simulink model "pedal_req_02"  (R2018b)
settings: Solver=FixedStepDiscrete  StartTime=0.0  StopTime=10.0  RelTol=1e-3
libraries: simulink x1
settings Model: Creator=yangbo  LastModifiedBy=yangbo_91
settings OptimizationCC: DefaultParameterBehavior=Inlined  EnhancedBackFolding=on  PassReuseOutputArgsAs=Individual arguments  OptimizeBlockOrder=speed  DifferentSizesBufferReuse=on  OptimizationCustomize=off
settings DebuggingCC: ParameterTunabilityLossMsg=error
settings SFSimCC: MATLABDynamicMemAlloc=off
settings RTWCC: SystemTargetFile=ert.tlc  TemplateMakefile=ert_default_tmf  GenerateReport=on  IncludeHyperlinkInReport=on  LaunchReport=on  GenerateTraceInfo=on  GenerateTraceReport=on  GenerateTraceReportSl=on  GenerateTraceReportSf=on  GenerateTraceReportEml=on
settings CodeAppCC: ForceParamTrailComments=on  IgnoreCustomStorageClasses=off  OperatorAnnotations=on  SimulinkDataObjDesc=on  SFDataObjDesc=on  InsertBlockDesc=on
settings ERTTargetCC: TargetLangStandard=C99 (ISO)  GenerateSampleERTMain=on  InlinedParameterPlacement=NonHierarchical  ERTCustomFileTemplate=example_file_process.tlc

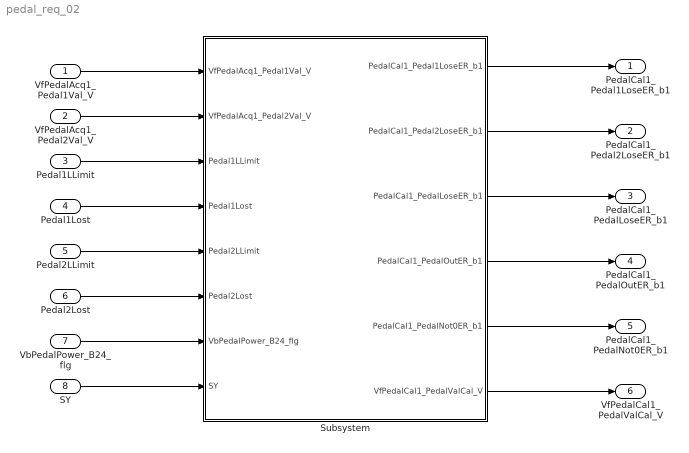
== system pedal_req_02 ==
  VfPedalAcq1_Pedal1Val_V : Inport
  VfPedalAcq1_Pedal2Val_V : Inport  Port=2
  Pedal1LLimit : Inport  Port=3
  Pedal1Lost : Inport  Port=4
  Pedal2LLimit : Inport  Port=5
  Pedal2Lost : Inport  Port=6
  VbPedalPower_B24_flg : Inport  Port=7
  SY : Inport  Port=8
  Subsystem : Subsystem  TreatAsAtomicUnit=on
  PedalCal1_Pedal1LoseER_b1 : Outport
  PedalCal1_Pedal2LoseER_b1 : Outport  Port=2
  PedalCal1_PedalLoseER_b1 : Outport  Port=3
  PedalCal1_PedalOutER_b1 : Outport  Port=4
  PedalCal1_PedalNot0ER_b1 : Outport  Port=5
  VfPedalCal1_PedalValCal_V : Outport  Port=6
  wires:
  VfPedalAcq1_Pedal1Val_V/1 -> Subsystem/1(VfPedalAcq1_Pedal1Val_V)
  VfPedalAcq1_Pedal2Val_V/1 -> Subsystem/2(VfPedalAcq1_Pedal2Val_V)
  Pedal1LLimit/1 -> Subsystem/3(Pedal1LLimit)
  Pedal1Lost/1 -> Subsystem/4(Pedal1Lost)
  Pedal2LLimit/1 -> Subsystem/5(Pedal2LLimit)
  Pedal2Lost/1 -> Subsystem/6(Pedal2Lost)
  VbPedalPower_B24_flg/1 -> Subsystem/7(VbPedalPower_B24_flg)
  SY/1 -> Subsystem/8(SY)
  Subsystem/1(PedalCal1_Pedal1LoseER_b1) -> PedalCal1_Pedal1LoseER_b1/1
  Subsystem/2(PedalCal1_Pedal2LoseER_b1) -> PedalCal1_Pedal2LoseER_b1/1
  Subsystem/3(PedalCal1_PedalLoseER_b1) -> PedalCal1_PedalLoseER_b1/1
  Subsystem/4(PedalCal1_PedalOutER_b1) -> PedalCal1_PedalOutER_b1/1
  Subsystem/5(PedalCal1_PedalNot0ER_b1) -> PedalCal1_PedalNot0ER_b1/1
  Subsystem/6(VfPedalCal1_PedalValCal_V) -> VfPedalCal1_PedalValCal_V/1

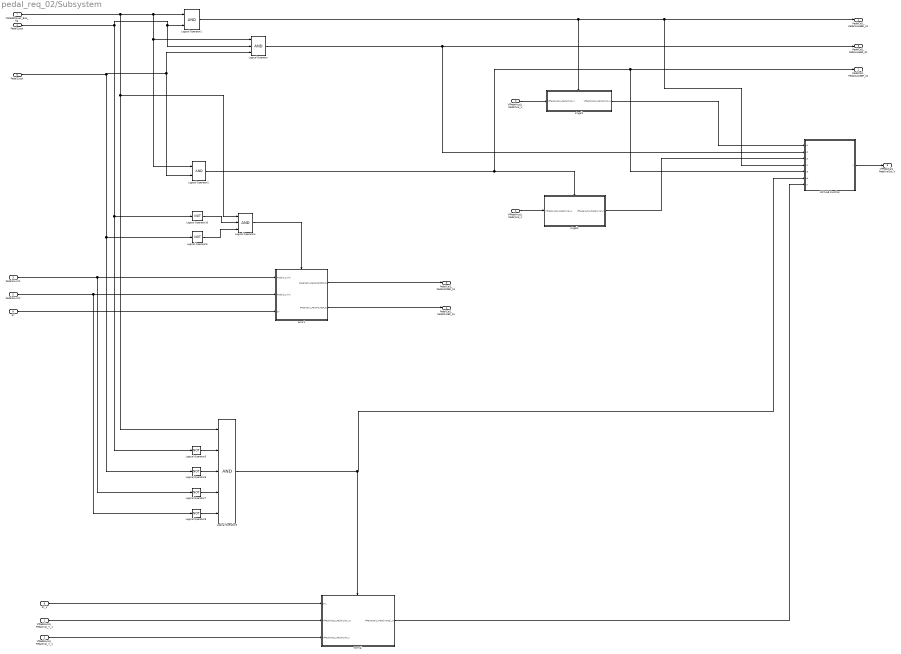
== system pedal_req_02/Subsystem ==
  VfPedalAcq1_Pedal1Val_V : Inport
  VfPedalAcq1_Pedal2Val_V : Inport  Port=2
  Pedal1LLimit : Inport  Port=3
  Pedal1Lost : Inport  Port=4
  Pedal2LLimit : Inport  Port=5
  Pedal2Lost : Inport  Port=6
  VbPedalPower_B24_flg : Inport  Port=7
  SY : Inport  Port=8
  Logical Operator : Logic  Inputs=3  AllPortsSameDT=off  OutDataTypeStr=boolean
  Logical Operator1 : Logic  AllPortsSameDT=off  OutDataTypeStr=boolean
  Logical Operator10 : Logic  Operator=NOT  Inputs=3  AllPortsSameDT=off  OutDataTypeStr=boolean
  Logical Operator2 : Logic  AllPortsSameDT=off  OutDataTypeStr=boolean
  Logical Operator3 : Logic  Inputs=5  AllPortsSameDT=off  OutDataTypeStr=boolean
  Logical Operator4 : Logic  Inputs=3  AllPortsSameDT=off  OutDataTypeStr=boolean
  Logical Operator{5..8} (4 alike) : Logic  Operator=NOT  AllPortsSameDT=off  OutDataTypeStr=boolean
  Logical Operator9 : Logic  Operator=NOT  Inputs=3  AllPortsSameDT=off  OutDataTypeStr=boolean
  MATLAB Function : MATLAB Function  TreatAsAtomicUnit=on
  SY_1 : InportShadow  Port=8
  VfPedalAcq1_Pedal1Val_V_1 : InportShadow
  VfPedalAcq1_Pedal2Val_V_1 : InportShadow  Port=2
  error1 : Subsystem  TreatAsAtomicUnit=on
  normal : Subsystem  TreatAsAtomicUnit=on
  singal1 : Subsystem  TreatAsAtomicUnit=on
  singal2 : Subsystem  TreatAsAtomicUnit=on
  PedalCal1_Pedal1LoseER_b1 : Outport
  PedalCal1_Pedal2LoseER_b1 : Outport  Port=2
  PedalCal1_PedalLoseER_b1 : Outport  Port=3
  PedalCal1_PedalOutER_b1 : Outport  Port=4
  PedalCal1_PedalNot0ER_b1 : Outport  Port=5
  VfPedalCal1_PedalValCal_V : Outport  Port=6
  wires:
  VbPedalPower_B24_flg/1 -> Logical Operator4/1, Logical Operator3/1, Logical Operator/1, Logical Operator2/1, Logical Operator1/1
  Pedal1LLimit/1 -> Logical Operator7/1, error1/1(Pedal1LLimit)
  SY/1 -> error1/3(SY)
  Logical Operator1/1 -> PedalCal1_Pedal1LoseER_b1/1, MATLAB Function/4(u4), singal1/Enable
  Logical Operator9/1 -> Logical Operator4/3
  Pedal2Lost/1 -> Logical Operator2/2, Logical Operator/3, Logical Operator9/1, Logical Operator6/1
  error1/1(PedalCal1_PedalNot0ER_b1) -> PedalCal1_PedalNot0ER_b1/1
  Pedal1Lost/1 -> Logical Operator/2, Logical Operator1/2, Logical Operator10/1, Logical Operator5/1
  VfPedalAcq1_Pedal1Val_V_1/1 -> normal/2(VfPedalAcq1_Pedal1Val_V1)
  Pedal2LLimit/1 -> Logical Operator8/1, error1/2(Pedal2LLimit)
  VfPedalAcq1_Pedal1Val_V/1 -> singal2/1(VfPedalAcq1_Pedal1Val_V)
  Logical Operator10/1 -> Logical Operator4/2
  Logical Operator4/1 -> error1/Enable
  Logical Operator2/1 -> PedalCal1_Pedal2LoseER_b1/1, MATLAB Function/5(u5), singal2/Enable
  singal2/1(VfPedalAcq1_Pedal1Val_V_) -> MATLAB Function/3(u3)
  singal1/1(VfPedalAcq1_Pedal2Val_V_) -> MATLAB Function/1(u1)
  Logical Operator5/1 -> Logical Operator3/2
  error1/2(PedalCal1_PedalOutER_b1) -> PedalCal1_PedalOutER_b1/1
  Logical Operator3/1 -> MATLAB Function/6(u6), normal/Enable
  Logical Operator/1 -> PedalCal1_PedalLoseER_b1/1, MATLAB Function/2(u2)
  Logical Operator8/1 -> Logical Operator3/5
  VfPedalAcq1_Pedal2Val_V_1/1 -> normal/3(VfPedalAcq1_Pedal2Val_V)
  SY_1/1 -> normal/1(SY1)
  VfPedalAcq1_Pedal2Val_V/1 -> singal1/1(VfPedalAcq1_Pedal2Val_V)
  Logical Operator7/1 -> Logical Operator3/4
  MATLAB Function/1(y) -> VfPedalCal1_PedalValCal_V/1
  normal/1(VfPedalCal1_PedalValCal_V1) -> MATLAB Function/7(u7)
  Logical Operator6/1 -> Logical Operator3/3

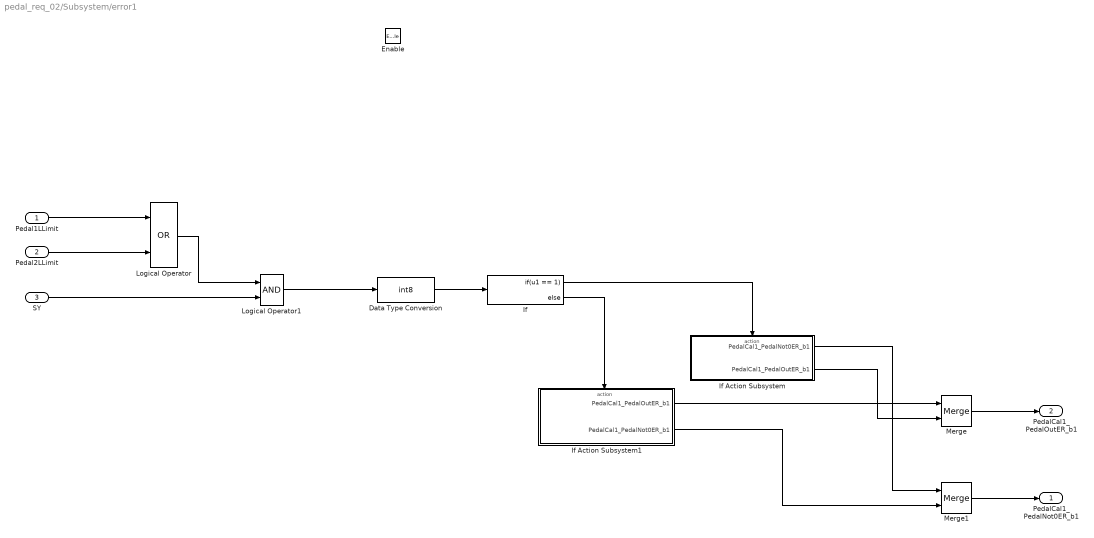
== system pedal_req_02/Subsystem/error1 ==
  Pedal1LLimit : Inport
  Pedal2LLimit : Inport  Port=2
  SY : Inport  Port=3
  Enable : EnablePort
  Data Type Conversion : DataTypeConversion  OutDataTypeStr=int8
  If : If  IfExpression=u1 == 1
  If Action Subsystem : Subsystem  TreatAsAtomicUnit=on
  If Action Subsystem1 : Subsystem  TreatAsAtomicUnit=on
  Logical Operator : Logic  Operator=OR  AllPortsSameDT=off  OutDataTypeStr=boolean
  Logical Operator1 : Logic  AllPortsSameDT=off  OutDataTypeStr=boolean
  Merge : Merge
  Merge1 : Merge
  PedalCal1_PedalNot0ER_b1 : Outport
  PedalCal1_PedalOutER_b1 : Outport  Port=2
  wires:
  Pedal1LLimit/1 -> Logical Operator/1
  Pedal2LLimit/1 -> Logical Operator/2
  Logical Operator/1 -> Logical Operator1/1
  Data Type Conversion/1 -> If/1
  If/1 -> If Action Subsystem/Action
  If/2 -> If Action Subsystem1/Action
  SY/1 -> Logical Operator1/2
  Logical Operator1/1 -> Data Type Conversion/1
  If Action Subsystem1/1(PedalCal1_PedalOutER_b1) -> Merge/1
  If Action Subsystem/1(PedalCal1_PedalNot0ER_b1) -> Merge1/1
  If Action Subsystem/2(PedalCal1_PedalOutER_b1) -> Merge/2
  Merge/1 -> PedalCal1_PedalOutER_b1/1
  If Action Subsystem1/2(PedalCal1_PedalNot0ER_b1) -> Merge1/2
  Merge1/1 -> PedalCal1_PedalNot0ER_b1/1

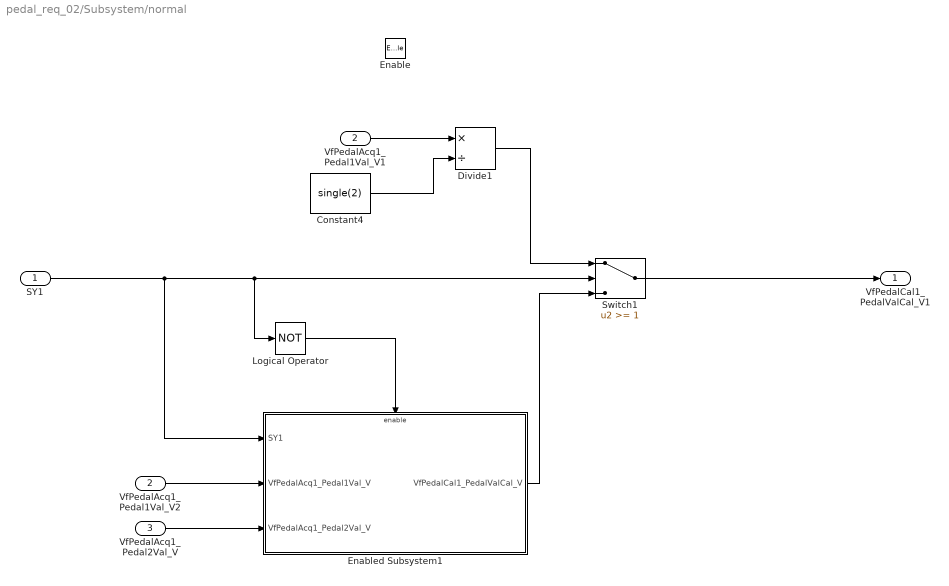
== system pedal_req_02/Subsystem/normal ==
  SY1 : Inport
  VfPedalAcq1_Pedal1Val_V1 : Inport  Port=2
  VfPedalAcq1_Pedal2Val_V : Inport  Port=3
  Enable : EnablePort
  Constant4 : Constant  Value=single(2)
  Divide1 : Product  Inputs=*/
  Enabled Subsystem1 : Subsystem  TreatAsAtomicUnit=on
  Logical Operator : Logic  Operator=NOT  AllPortsSameDT=off  OutDataTypeStr=boolean
  Switch1 : Switch  Threshold=1
  VfPedalAcq1_Pedal1Val_V2 : InportShadow  Port=2
  VfPedalCal1_PedalValCal_V1 : Outport
  wires:
  SY1/1 -> Enabled Subsystem1/1(SY1), Logical Operator/1, Switch1/2
  Switch1/1 -> VfPedalCal1_PedalValCal_V1/1
  VfPedalAcq1_Pedal1Val_V1/1 -> Divide1/1
  Constant4/1 -> Divide1/2
  Divide1/1 -> Switch1/1
  Enabled Subsystem1/1(VfPedalCal1_PedalValCal_V) -> Switch1/3
  VfPedalAcq1_Pedal2Val_V/1 -> Enabled Subsystem1/3(VfPedalAcq1_Pedal2Val_V)
  VfPedalAcq1_Pedal1Val_V2/1 -> Enabled Subsystem1/2(VfPedalAcq1_Pedal1Val_V)
  Logical Operator/1 -> Enabled Subsystem1/Enable

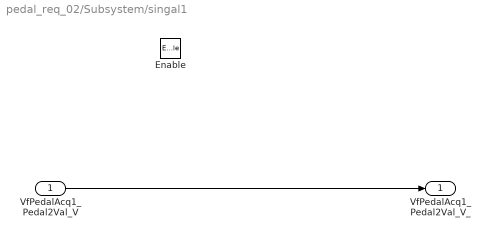
== system pedal_req_02/Subsystem/singal1 ==
  VfPedalAcq1_Pedal2Val_V : Inport
  Enable : EnablePort
  VfPedalAcq1_Pedal2Val_V_ : Outport
  wires:
  VfPedalAcq1_Pedal2Val_V/1 -> VfPedalAcq1_Pedal2Val_V_/1

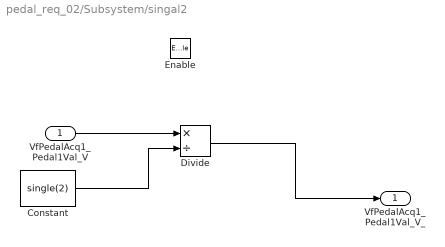
== system pedal_req_02/Subsystem/singal2 ==
  VfPedalAcq1_Pedal1Val_V : Inport
  Enable : EnablePort
  Constant : Constant  Value=single(2)
  Divide : Product  Inputs=*/
  VfPedalAcq1_Pedal1Val_V_ : Outport
  wires:
  VfPedalAcq1_Pedal1Val_V/1 -> Divide/1
  Constant/1 -> Divide/2
  Divide/1 -> VfPedalAcq1_Pedal1Val_V_/1

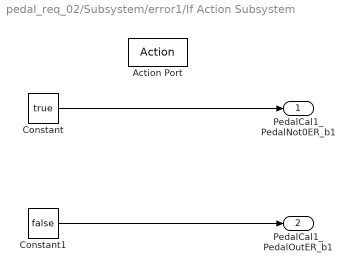
== system pedal_req_02/Subsystem/error1/If Action Subsystem ==
  Action Port : ActionPort  ActionType=then
  Constant : Constant  Value=true
  Constant1 : Constant  Value=false
  PedalCal1_PedalNot0ER_b1 : Outport
  PedalCal1_PedalOutER_b1 : Outport  Port=2
  wires:
  Constant/1 -> PedalCal1_PedalNot0ER_b1/1
  Constant1/1 -> PedalCal1_PedalOutER_b1/1

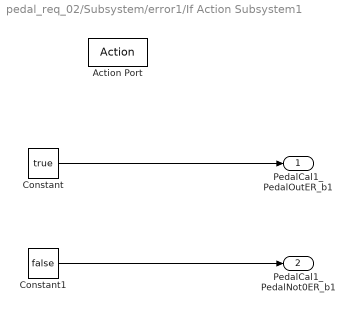
== system pedal_req_02/Subsystem/error1/If Action Subsystem1 ==
  Action Port : ActionPort  ActionType=else
  Constant : Constant  Value=true
  Constant1 : Constant  Value=false
  PedalCal1_PedalOutER_b1 : Outport
  PedalCal1_PedalNot0ER_b1 : Outport  Port=2
  wires:
  Constant/1 -> PedalCal1_PedalOutER_b1/1
  Constant1/1 -> PedalCal1_PedalNot0ER_b1/1

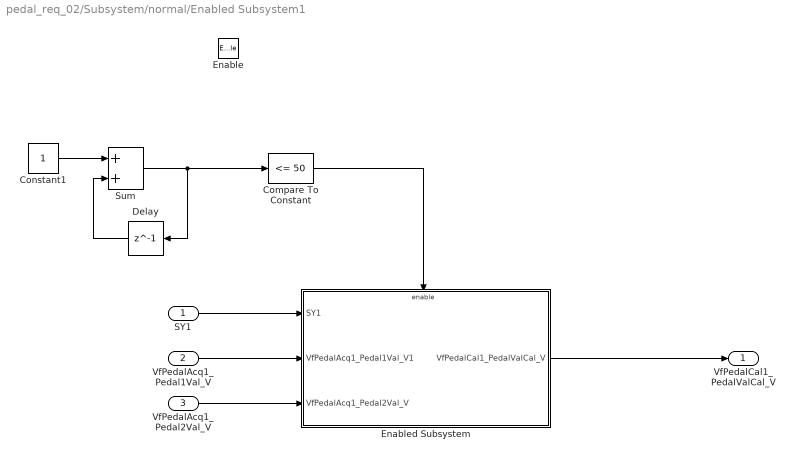
== system pedal_req_02/Subsystem/normal/Enabled Subsystem1 ==
  SY1 : Inport
  VfPedalAcq1_Pedal1Val_V : Inport  Port=2
  VfPedalAcq1_Pedal2Val_V : Inport  Port=3
  Enable : EnablePort
  Compare To Constant : simulink/Logic and Bit Operations/Compare To Constant  relop=<=  const=50  OutDataTypeStr=boolean
  Constant1 : Constant
  Delay : Delay  DelayLength=1  InitialCondition=0
  Enabled Subsystem : Subsystem  TreatAsAtomicUnit=on
  Sum : Sum
  VfPedalCal1_PedalValCal_V : Outport
  wires:
  Constant1/1 -> Sum/1
  Sum/1 -> Delay/1, Compare To Constant/1
  Delay/1 -> Sum/2
  Compare To Constant/1 -> Enabled Subsystem/Enable
  SY1/1 -> Enabled Subsystem/1(SY1)
  VfPedalAcq1_Pedal1Val_V/1 -> Enabled Subsystem/2(VfPedalAcq1_Pedal1Val_V1)
  VfPedalAcq1_Pedal2Val_V/1 -> Enabled Subsystem/3(VfPedalAcq1_Pedal2Val_V)
  Enabled Subsystem/1(VfPedalCal1_PedalValCal_V) -> VfPedalCal1_PedalValCal_V/1

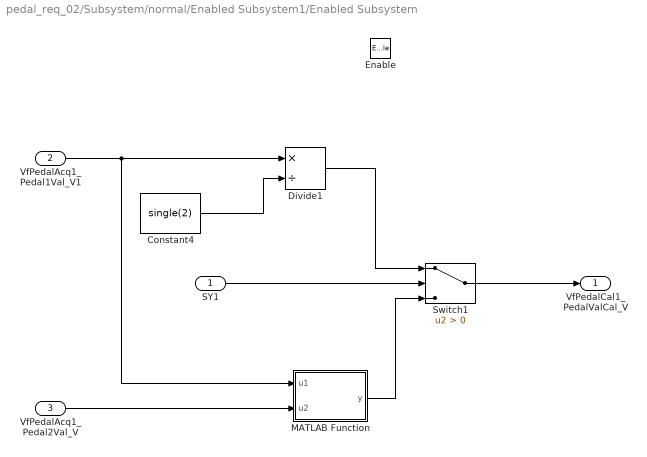
== system pedal_req_02/Subsystem/normal/Enabled Subsystem1/Enabled Subsystem ==
  SY1 : Inport
  VfPedalAcq1_Pedal1Val_V1 : Inport  Port=2
  VfPedalAcq1_Pedal2Val_V : Inport  Port=3
  Enable : EnablePort
  Constant4 : Constant  Value=single(2)
  Divide1 : Product  Inputs=*/
  MATLAB Function : MATLAB Function  TreatAsAtomicUnit=on
  Switch1 : Switch  Criteria=u2 > Threshold
  VfPedalCal1_PedalValCal_V : Outport
  wires:
  SY1/1 -> Switch1/2
  Switch1/1 -> VfPedalCal1_PedalValCal_V/1
  VfPedalAcq1_Pedal1Val_V1/1 -> MATLAB Function/1(u1), Divide1/1
  Constant4/1 -> Divide1/2
  Divide1/1 -> Switch1/1
  VfPedalAcq1_Pedal2Val_V/1 -> MATLAB Function/2(u2)
  MATLAB Function/1(y) -> Switch1/3

== matlab function pedal_req_02/Subsystem/MATLAB Function ==
  data: u1 input; y output; u2 input; u3 input; u4 input; u5 input; u6 input; u7 input
function y = fcn(u1,u2,u3,u4,u5,u6,u7)
%#codegen
if(u2==1)
    y=0;
elseif(u4==1)
    y=u1;
elseif(u5==1)
    y=u3;
elseif(u6==1)
    y=u7;
else
    y=0;
end

== matlab function pedal_req_02/Subsystem/normal/Enabled Subsystem1/Enabled Subsystem/MATLAB Function ==
  data: u1 input; y output; u2 input
function y = fcn(u1,u2)
%#codegen
u12=u1/2;
if(u12>u2)
    y=u2;
else
    y=u12;
end
